simulink model "robot"  (R2025b)
settings: Solver=VariableStepAuto  StartTime=0.0  StopTime=16  RelTol=1e-3
undefined symbols (not defined in the file or in its folder): Kd_dist, Kd_head, Ki_dist, Ki_head, Kp_dist, Kp_head
libraries: slpidlib x2
settings Model: Creator=cyc  LastModifiedBy=cyc

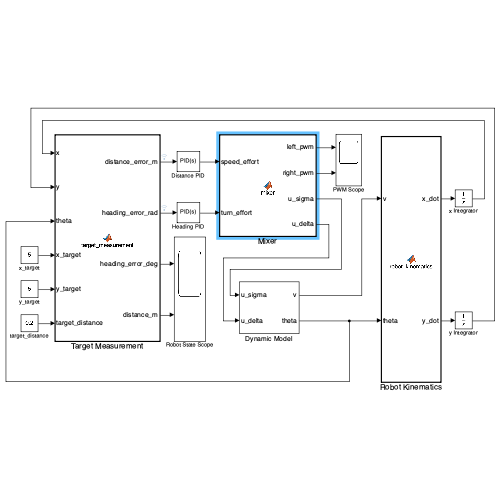
[thumbnail: Simulink's stored preview of the top-level diagram]
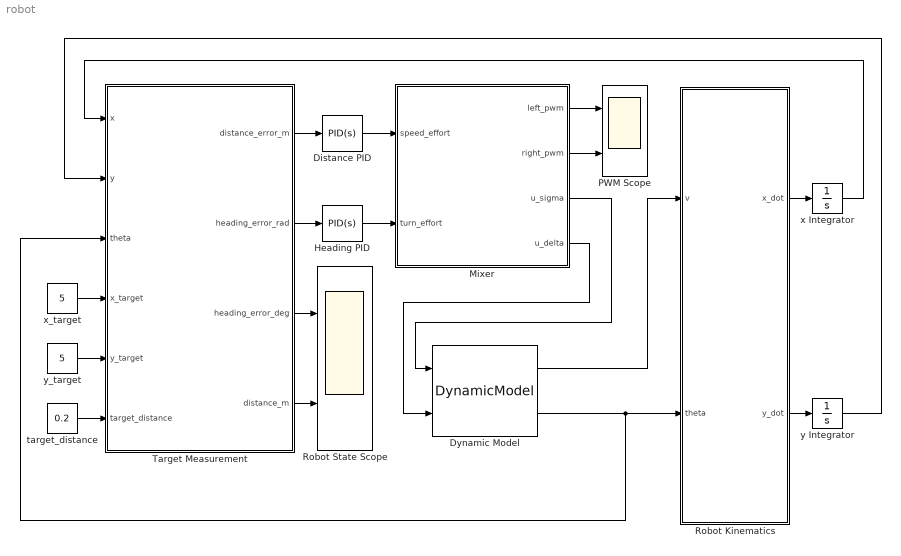
== system robot ==
  Distance PID : slpidlib/PID Controller  Controller=PID  Form=Parallel  TimeDomain=Continuous-time  UseExternalTs=off  SampleTime=-1  IntegratorMethod=Forward Euler  FilterMethod=Forward Euler  ControllerParametersSource=internal  P=Kp_dist  I=Ki_dist  UseKiTs=off  D=Kd_dist  UseExternalDerivativeSource=off  N=100  UseFilter=on  TunerSelectOption=Transfer Function Based (PID Tuner App)  InitialConditionSource=internal  InitialConditionForIntegrator=0  InitialConditionForFilter=0  DifferentiatorICPrevScaledInput=0  ExternalReset=none  TrackingMode=off  Kt=1  LimitOutput=off  SatLimitsSource=internal  UpperSaturationLimit=inf  LowerSaturationLimit=-inf  LinearizeAsGain=on  AntiWindupMode=none  Kb=1  LimitIntegrator=off  UpperIntegratorSaturationLimit=inf  LowerIntegratorSaturationLimit=-inf  POutMin=[]  POutMax=[]  IOutMin=[]  IOutMax=[]  DOutMin=[]  DOutMax=[]  NOutMin=[]  NOutMax=[]  SumOutMin=[]  SumOutMax=[]  SaturationOutMin=[]  SaturationOutMax=[]  PParamMin=[]  PParamMax=[]  IParamMin=[]  IParamMax=[]  DParamMin=[]  DParamMax=[]  NParamMin=[]  NParamMax=[]  KbParamMin=[]  KbParamMax=[]  KtParamMin=[]  KtParamMax=[]  KbOutMin=[]  KbOutMax=[]  KtOutMin=[]  KtOutMax=[]  IntegratorOutMin=[]  IntegratorOutMax=[]  FilterOutMin=[]  FilterOutMax=[]  SumI1OutMin=[]  SumI1OutMax=[]  SumI2OutMin=[]  SumI2OutMax=[]  SumI3OutMin=[]  SumI3OutMax=[]  SumI4OutMin=[]  SumI4OutMax=[]  SumDOutMin=[]  SumDOutMax=[]  DifferentiatorOutMin=[]  DifferentiatorOutMax=[]  FilterDiffOutCoefMin=[]  FilterDiffOutCoefMax=[]  ReciprocalOutMin=[]  ReciprocalOutMax=[]  SumDenOutMin=[]  SumDenOutMax=[]  SumNumOutMin=[]  SumNumOutMax=[]  DivideOutMin=[]  DivideOutMax=[]  UdiffTsProdOutMin=[]  UdiffTsProdOutMax=[]  NTsProdOutMin=[]  NTsProdOutMax=[]  UintegralTsProdOutMin=[]  UintegralTsProdOutMax=[]  UngainTsProdOutMin=[]  UngainTsProdOutMax=[]  ClampingZeroOutDataTypeStr=Inherit: Inherit via back propagation  ClampingZeroOutMin=[]  ClampingZeroOutMax=[]  FilterDenConstantOutDataTypeStr=Inherit: Inherit via back propagation  FilterDenConstantOutMin=[]  FilterDenConstantOutMax=[]  PCopyOutDataTypeStr=Inherit: Inherit via back propagation  PCopyOutMin=[]  PCopyOutMax=[]  NCopyOutDataTypeStr=Inherit: Inherit via back propagation  NCopyOutMin=[]  NCopyOutMax=[]  IntegratorContinuousStateAttributes=''  IntegratorStateMustResolveToSignalObject=off  IntegratorRTWStateStorageClass=Auto  FilterContinuousStateAttributes=''  FilterStateMustResolveToSignalObject=off  FilterRTWStateStorageClass=Auto  ParallelPVariant=InternalParameters  IdealPVariant=Disabled  IVariant=InternalParameters  DVariant=InternalParameters  IntegratorVariant=Continuous  SatVariant=Disabled  AWVariant=Passthrough  PCopyVariant=Disabled  TRVariant=Disabled  FdbkBlocksVariant=Forward  IdealPFdbkVariant=Disabled  SatFdbkVariant=Disabled  DerivativeFilterVariant=ContFilter  NVariant=InternalParameters  NCopyVariant=Disabled  FilterICVariant=InternalICsFilter  IntegratorICVariant=InternalICs  ExternalResetVariant=Disabled  TRSumVariant=Passthrough  SumFdbkVariant=Disabled  SumVariant=Sum_PID  TsampFilterVariant=InternalTs  TsampNgainVariant=Passthrough  TsampIntegralVariant=Disabled_SignalSpec  ExternalSaturationOutDataTypeStr=Inherit: Same as second input  DerivativeSourceVariant=ErrorSignal  PreIntVariant=InternalPreInt
  Dynamic Model : M-S-Function  FunctionName=DynamicModel
      mask Display:
      | port_label('input', 1, 'u_sigma');
      | port_label('input', 2, 'u_delta');
      | 
      | port_label('output', 1, 'v');
      | port_label('output', 2, 'theta');
  Heading PID : slpidlib/PID Controller  Controller=PID  Form=Parallel  TimeDomain=Continuous-time  UseExternalTs=off  SampleTime=-1  IntegratorMethod=Forward Euler  FilterMethod=Forward Euler  ControllerParametersSource=internal  P=Kp_head  I=Ki_head  UseKiTs=off  D=Kd_head  UseExternalDerivativeSource=off  N=100  UseFilter=on  TunerSelectOption=Transfer Function Based (PID Tuner App)  InitialConditionSource=internal  InitialConditionForIntegrator=0  InitialConditionForFilter=0  DifferentiatorICPrevScaledInput=0  ExternalReset=none  TrackingMode=off  Kt=1  LimitOutput=off  SatLimitsSource=internal  UpperSaturationLimit=inf  LowerSaturationLimit=-inf  LinearizeAsGain=on  AntiWindupMode=none  Kb=1  LimitIntegrator=off  UpperIntegratorSaturationLimit=inf  LowerIntegratorSaturationLimit=-inf  POutMin=[]  POutMax=[]  IOutMin=[]  IOutMax=[]  DOutMin=[]  DOutMax=[]  NOutMin=[]  NOutMax=[]  SumOutMin=[]  SumOutMax=[]  SaturationOutMin=[]  SaturationOutMax=[]  PParamMin=[]  PParamMax=[]  IParamMin=[]  IParamMax=[]  DParamMin=[]  DParamMax=[]  NParamMin=[]  NParamMax=[]  KbParamMin=[]  KbParamMax=[]  KtParamMin=[]  KtParamMax=[]  KbOutMin=[]  KbOutMax=[]  KtOutMin=[]  KtOutMax=[]  IntegratorOutMin=[]  IntegratorOutMax=[]  FilterOutMin=[]  FilterOutMax=[]  SumI1OutMin=[]  SumI1OutMax=[]  SumI2OutMin=[]  SumI2OutMax=[]  SumI3OutMin=[]  SumI3OutMax=[]  SumI4OutMin=[]  SumI4OutMax=[]  SumDOutMin=[]  SumDOutMax=[]  DifferentiatorOutMin=[]  DifferentiatorOutMax=[]  FilterDiffOutCoefMin=[]  FilterDiffOutCoefMax=[]  ReciprocalOutMin=[]  ReciprocalOutMax=[]  SumDenOutMin=[]  SumDenOutMax=[]  SumNumOutMin=[]  SumNumOutMax=[]  DivideOutMin=[]  DivideOutMax=[]  UdiffTsProdOutMin=[]  UdiffTsProdOutMax=[]  NTsProdOutMin=[]  NTsProdOutMax=[]  UintegralTsProdOutMin=[]  UintegralTsProdOutMax=[]  UngainTsProdOutMin=[]  UngainTsProdOutMax=[]  ClampingZeroOutDataTypeStr=Inherit: Inherit via back propagation  ClampingZeroOutMin=[]  ClampingZeroOutMax=[]  FilterDenConstantOutDataTypeStr=Inherit: Inherit via back propagation  FilterDenConstantOutMin=[]  FilterDenConstantOutMax=[]  PCopyOutDataTypeStr=Inherit: Inherit via back propagation  PCopyOutMin=[]  PCopyOutMax=[]  NCopyOutDataTypeStr=Inherit: Inherit via back propagation  NCopyOutMin=[]  NCopyOutMax=[]  IntegratorContinuousStateAttributes=''  IntegratorStateMustResolveToSignalObject=off  IntegratorRTWStateStorageClass=Auto  FilterContinuousStateAttributes=''  FilterStateMustResolveToSignalObject=off  FilterRTWStateStorageClass=Auto  ParallelPVariant=InternalParameters  IdealPVariant=Disabled  IVariant=InternalParameters  DVariant=InternalParameters  IntegratorVariant=Continuous  SatVariant=Disabled  AWVariant=Passthrough  PCopyVariant=Disabled  TRVariant=Disabled  FdbkBlocksVariant=Forward  IdealPFdbkVariant=Disabled  SatFdbkVariant=Disabled  DerivativeFilterVariant=ContFilter  NVariant=InternalParameters  NCopyVariant=Disabled  FilterICVariant=InternalICsFilter  IntegratorICVariant=InternalICs  ExternalResetVariant=Disabled  TRSumVariant=Passthrough  SumFdbkVariant=Disabled  SumVariant=Sum_PID  TsampFilterVariant=InternalTs  TsampNgainVariant=Passthrough  TsampIntegralVariant=Disabled_SignalSpec  ExternalSaturationOutDataTypeStr=Inherit: Same as second input  DerivativeSourceVariant=ErrorSignal  PreIntVariant=InternalPreInt
  Mixer : MATLAB Function  TreatAsAtomicUnit=on
  PWM Scope : Scope  NumInputPorts=2
      settings: ActiveDisplayYMinimum=-18.749999999999996  ActiveDisplayYMaximum=168.75
  Robot Kinematics : MATLAB Function  TreatAsAtomicUnit=on
  Robot State Scope : Scope  NumInputPorts=2
      settings: ActiveDisplayYMinimum=-5.6883101048853728  ActiveDisplayYMaximum=50.632034456098374
  Target Measurement : MATLAB Function  TreatAsAtomicUnit=on
  target_distance : Constant  Value=0.2
  x Integrator : Integrator
  x_target : Constant  Value=5
  y Integrator : Integrator
  y_target : Constant  Value=5
  wires:
  Robot Kinematics/1(x_dot) -> x Integrator/1
  Distance PID/1 -> Mixer/1(speed_effort)
  Heading PID/1 -> Mixer/2(turn_effort)
  Target Measurement/2(heading_error_rad) -> Heading PID/1
  y Integrator/1 -> Target Measurement/2(y)
  Dynamic Model/2 -> Robot Kinematics/2(theta), Target Measurement/3(theta)
  Target Measurement/1(distance_error_m) -> Distance PID/1
  Robot Kinematics/2(y_dot) -> y Integrator/1
  x Integrator/1 -> Target Measurement/1(x)
  x_target/1 -> Target Measurement/4(x_target)
  y_target/1 -> Target Measurement/5(y_target)
  target_distance/1 -> Target Measurement/6(target_distance)
  Target Measurement/3(heading_error_deg) -> Robot State Scope/1
  Target Measurement/4(distance_m) -> Robot State Scope/2
  Mixer/2(right_pwm) -> PWM Scope/2
  Mixer/1(left_pwm) -> PWM Scope/1
  Dynamic Model/1 -> Robot Kinematics/1(v)
  Mixer/3(u_sigma) -> Dynamic Model/1
  Mixer/4(u_delta) -> Dynamic Model/2

== matlab function robot/Mixer ==
  data: speed_effort input; left_pwm output; turn_effort input; right_pwm output; u_sigma output; u_delta output
function [left_pwm, right_pwm, u_sigma, u_delta] = mixer(speed_effort, turn_effort)
% Matches raspberry/motor_mixer.py.
% speed_effort comes from distance PID.
% turn_effort comes from heading PID.
% left_pwm/right_pwm are Arduino commands.
% u_sigma/u_delta are effective plant inputs for the dynamic model.

max_pwm = 100;
min_pwm = 27;

max_speed_effort = 1.0;
max_turn_effort = 1.3;

turn_gain = 1.0;
pivot_turn_gain = 0.65;
pivot_speed_threshold = 0.05;

speed = clamp(speed_effort / max_speed_effort, -1.0, 1.0);
turn = clamp(turn_effort / max_turn_effort, -1.0, 1.0);

if abs(speed) < pivot_speed_threshold
    left = -turn * pivot_turn_gain;
    right = turn * pivot_turn_gain;
else
    left = speed - turn * turn_gain;
    right = speed + turn * turn_gain;
end

scale = max([1.0, abs(left), abs(right)]);
left = left / scale;
right = right / scale;

left_pwm = apply_pwm(left, min_pwm, max_pwm);
right_pwm = apply_pwm(right, min_pwm, max_pwm);

left_eff_pwm = effective_pwm(left_pwm, min_pwm);
right_eff_pwm = effective_pwm(right_pwm, min_pwm);

u_sigma = (left_eff_pwm + right_eff_pwm) / 2.0;
u_delta = (right_eff_pwm - left_eff_pwm) / 2.0;
end


function y = clamp(x, lo, hi)
y = min(max(x, lo), hi);
end


function pwm = apply_pwm(value, min_pwm, max_pwm)
pwm = round(value * max_pwm);

if pwm == 0
    pwm = 0;
elseif abs(pwm) < min_pwm
    if pwm > 0
        pwm = min_pwm;
    else
        pwm = -min_pwm;
    end
end
end


function eff = effective_pwm(pwm, min_pwm)
if pwm > 0
    eff = pwm - min_pwm;
elseif pwm < 0
    eff = pwm + min_pwm;
else
    eff = 0;
end
end

== matlab function robot/Target Measurement ==
  data: x input; distance_error_m output; y input; theta input; x_target input; y_target input; target_distance input; heading_error_rad output; heading_error_deg output; distance_m output
function [distance_error_m, heading_error_rad, heading_error_deg, distance_m] = target_measurement(x, y, theta, x_target, y_target, target_distance)
% theta is robot heading in radians.
% x_target and y_target are fixed target coordinates in the world frame.

dx = x_target - x;
dy = y_target - y;

distance_m = sqrt(dx*dx + dy*dy);

target_angle = atan2(dy, dx);

heading_error_rad = target_angle - theta;
heading_error_rad = mod(heading_error_rad + pi, 2*pi) - pi;

heading_error_deg = heading_error_rad * 180.0 / pi;

distance_error_m = distance_m - target_distance;
end

== matlab function robot/Robot Kinematics ==
  data: v input; x_dot output; theta input; y_dot output
function [x_dot, y_dot] = robot_kinematics(v, theta)
% v: forward speed in m/s
% omega: angular speed in rad/s
% theta: robot heading in rad

x_dot = v * cos(theta);
y_dot = v * sin(theta);
end
